simulink model "ugv_ctrl_NEW"  (R2018a)
settings: Solver=VariableStepAuto  StartTime=0.0  StopTime=100000  FixedStep=0.00001  MaxStep=1  RelTol=1e-3
InitFcn:
  | ugv_parameters
undefined symbols (not defined in the file or in its folder): P, ugv_ctrl_encoders
settings Model: Creator=canla  LastModifiedBy=canla

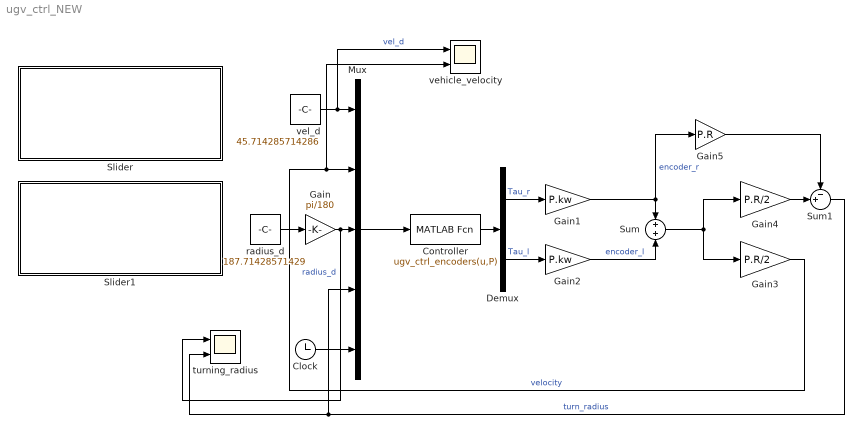
== system ugv_ctrl_NEW ==
  Clock : Clock
  Controller : MATLABFcn  MATLABFcn=ugv_ctrl_encoders(u,P)  OutputDimensions=2
  Demux : Demux  Outputs=2
  Gain : Gain  Gain=pi/180
  Gain1 : Gain  Gain=P.kw
  Gain2 : Gain  Gain=P.kw
  Gain3 : Gain  Gain=P.R/2
  Gain4 : Gain  Gain=P.R/2
  Gain5 : Gain  Gain=P.R
  Mux : Mux  Inputs=5
  Slider : Subsystem  DialogController=hmiCreateDDGDialog  IsWebBlock=on  mask(MWDashboardBlock){webBlockId=dd34282a-0a0b-4475-a121-34d8978dbf91, webBlockType=slider, ShowInLibBrowser=on, ShowInitialText=on, HMISrcModelName=ugv_ctrl_NEW}
      mask prompts: webBlockId "WebBlock Id"; webBlockType "WebBlock Type"; HMISrcModelName "Source Model"
      mask help: SimulinkHMI:dialogs:SliderDialogDesc
      mask Help: helpview([docroot '/mapfiles/simulink.map'], 'hmi_slider')
      mask Display:
      | if strcmp(get_param(bdroot(gcb),'BlockDiagramType'), 'library')
      |     image([(matlabroot) '/toolbox/simulink/hmi/icons/Slider.png']);
      | end
  Slider1 : Subsystem  DialogController=hmiCreateDDGDialog  IsWebBlock=on  mask(MWDashboardBlock){webBlockId=82b03c1d-0a29-4a55-84b6-77e889991205, webBlockType=slider, ShowInLibBrowser=on, ShowInitialText=on, HMISrcModelName=ugv_ctrl_NEW}
      mask prompts: webBlockId "WebBlock Id"; webBlockType "WebBlock Type"; HMISrcModelName "Source Model"
      mask help: SimulinkHMI:dialogs:SliderDialogDesc
      mask Help: helpview([docroot '/mapfiles/simulink.map'], 'hmi_slider')
      mask Display:
      | if strcmp(get_param(bdroot(gcb),'BlockDiagramType'), 'library')
      |     image([(matlabroot) '/toolbox/simulink/hmi/icons/Slider.png']);
      | end
  Sum : Sum
  Sum1 : Sum  Inputs=-+|
  radius_d : Constant  Value=187.71428571429
  turning_radius : Scope  NumInputPorts=2
  vehicle_velocity : Scope  NumInputPorts=2
  vel_d : Constant  Value=45.714285714286
  wires:
  vel_d/1 -> vehicle_velocity/1, Mux/1  "vel_d"
  Mux/1 -> Controller/1
  Clock/1 -> Mux/5
  radius_d/1 -> Gain/1
  Gain/1 -> turning_radius/1, Mux/3  "radius_d"
  Controller/1 -> Demux/1
  Demux/1 -> Gain1/1  "Tau_r"
  Demux/2 -> Gain2/1  "Tau_l"
  Gain1/1 -> Gain5/1, Sum/1  "encoder_r"
  Gain2/1 -> Sum/2  "encoder_l"
  Sum/1 -> Gain4/1, Gain3/1
  Gain4/1 -> Sum1/2
  Gain5/1 -> Sum1/1
  Gain3/1 -> vehicle_velocity/2, Mux/2  "velocity"
  Sum1/1 -> turning_radius/2, Mux/4  "turn_radius"

== system ugv_ctrl_NEW/Slider ==

== system ugv_ctrl_NEW/Slider1 ==
